simulink subsystem "Rigid_Body_Dynamics_Subsystem"  (R2026a)
settings: Solver=VariableStepAuto
settings Model: Creator=Eeman Aleem  LastModifiedBy=Eeman Aleem

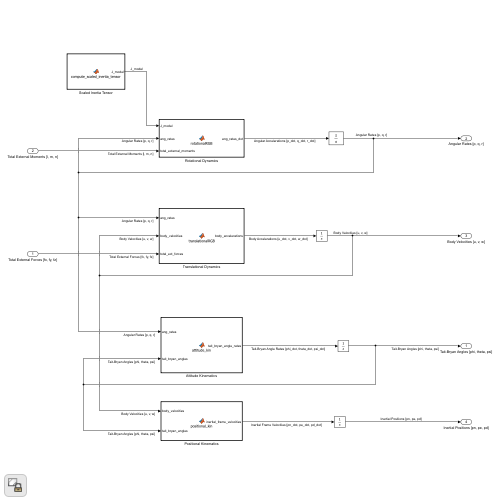
[thumbnail: Simulink's stored preview of the top-level diagram]
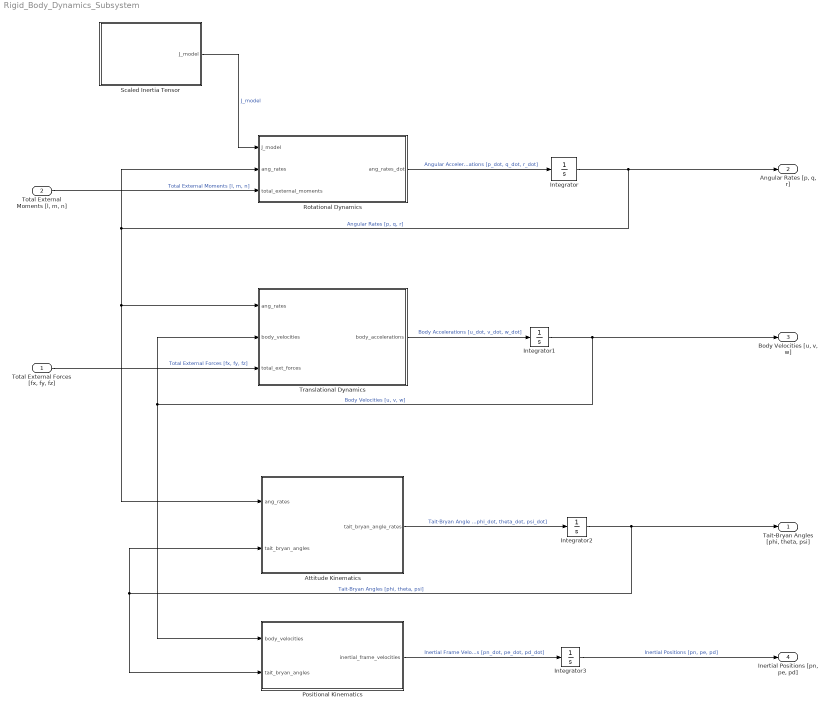
== system Rigid_Body_Dynamics_Subsystem ==
  "Total External Forces [fx, fy, fz]" : Inport
  "Total External Moments [l, m, n]" : Inport  Port=2
  Attitude Kinematics : MATLAB Function  TreatAsAtomicUnit=on
  Integrator{,1..3} (4 alike) : Integrator
  Positional Kinematics : MATLAB Function  TreatAsAtomicUnit=on
  Rotational Dynamics : MATLAB Function  TreatAsAtomicUnit=on
  Scaled Inertia Tensor : MATLAB Function  TreatAsAtomicUnit=on
  Translational Dynamics : MATLAB Function  TreatAsAtomicUnit=on
  "Tait-Bryan Angles [phi, theta, psi]" : Outport
  "Angular Rates [p, q, r]" : Outport  Port=2
  "Body Velocities [u, v, w]" : Outport  Port=3
  "Inertial Positions [pn, pe, pd]" : Outport  Port=4
  wires:
  Translational Dynamics/1(body_accelerations) -> Integrator1/1  "Body Accelerations [u_dot, v_dot, w_dot]"
  Positional Kinematics/1(inertial_frame_velocities) -> Integrator3/1  "Inertial Frame Velocities [pn_dot, pe_dot, pd_dot]"
  Rotational Dynamics/1(ang_rates_dot) -> Integrator/1  "Angular Accelerations [p_dot, q_dot, r_dot]"
  Attitude Kinematics/1(tait_bryan_angle_rates) -> Integrator2/1  "Tait-Bryan Angle Rates [phi_dot, theta_dot, psi_dot]"
  "Total External Moments [l, m, n]"/1 -> Rotational Dynamics/3(total_external_moments)  "Total External Moments [l, m, n]"
  Integrator3/1 -> "Inertial Positions [pn, pe, pd]"/1  "Inertial Positions [pn, pe, pd]"
  Integrator/1 -> Attitude Kinematics/1(ang_rates), Translational Dynamics/1(ang_rates), Rotational Dynamics/2(ang_rates), "Angular Rates [p, q, r]"/1  "Angular Rates [p, q, r]"
  Scaled Inertia Tensor/1(J_model) -> Rotational Dynamics/1(J_model)  "J_model"
  Integrator2/1 -> Attitude Kinematics/2(tait_bryan_angles), Positional Kinematics/2(tait_bryan_angles), "Tait-Bryan Angles [phi, theta, psi]"/1  "Tait-Bryan Angles [phi, theta, psi]"
  "Total External Forces [fx, fy, fz]"/1 -> Translational Dynamics/3(total_ext_forces)  "Total External Forces [fx, fy, fz]"
  Integrator1/1 -> Positional Kinematics/1(body_velocities), Translational Dynamics/2(body_velocities), "Body Velocities [u, v, w]"/1  "Body Velocities [u, v, w]"

== matlab function Rigid_Body_Dynamics_Subsystem/Rotational Dynamics ==
  data: J_model input size=[1 4]; ang_rates input size=[1 3]; ang_rates_dot output size=[1 3]; total_external_moments input size=[1 3]
function ang_rates_dot = rotationalRGB(J_model, ang_rates, total_external_moments)
    
    % Clarifying vars used
    Jx = J_model(1);
    Jy = J_model(2);
    Jz = J_model(3);
    Jxz = J_model(4);
    p = ang_rates(1);
    q = ang_rates(2);
    r = ang_rates(3);
    l = total_external_moments(1);
    m = total_external_moments(2);
    n = total_external_moments(3);
    
    % Calculate gamma constants from Equation 9
    Gamma = Jx * Jz - Jxz^2;
    Gamma1 = (Jxz * (Jx - Jy + Jz)) / Gamma;
    Gamma2 = ((Jz * (Jz - Jy)) + Jxz^2) / Gamma;
    Gamma3 = Jz / Gamma;
    Gamma4 = Jxz / Gamma;
    Gamma5 = (Jz - Jx) / Jy;
    Gamma6 = Jxz / Jy;
    Gamma7 = ((Jx * (Jx - Jy)) + Jxz^2) / Gamma;
    Gamma8 = Jx / Gamma;
    
    % Equation 9
    p_dot = Gamma1*p*q - Gamma2*q*r + Gamma3*l + Gamma4*n;
    q_dot = Gamma5*p*r - Gamma6*(p^2 - r^2) + (1/Jy)*m;
    r_dot = Gamma7*p*q - Gamma1*q*r + Gamma4*l + Gamma8*n;
    
    ang_rates_dot = [p_dot, q_dot, r_dot];

end

== matlab function Rigid_Body_Dynamics_Subsystem/Scaled Inertia Tensor ==
  data: J_model output size=[1 4]
function J_model = compute_scaled_inertia_tensor()
% This function calculates the scaled-down inertias for a model aircraft.
% It converts full-scale imperial inertias to SI units and applies a scaling factor.
%
% INPUTS:
%   J_fs array:
%       - Jx_full:   Full-scale roll inertia [slug·ft²]
%       - Jy_full:   Full-scale pitch inertia [slug·ft²]
%       - Jz_full:   Full-scale yaw inertia [slug·ft²]
%       - Jxz_full:  Full-scale product of inertia [slug·ft²]
%   mass array:
%       - m_full:    Full-scale aircraft mass [kg]
%       - m_model:   Model aircraft mass [kg]
%   gsf: Geometric scale factor
%
% OUTPUTS:
%   Jx: Scaled model roll inertia [kg·m²]
%   Jy: Scaled model pitch inertia [kg·m²]
%   Jz: Scaled model yaw inertia [kg·m²]
%   Jxz: Scaled model product of inertia [kg·m²]

% Input Constants:
m_model = GeoConsts.m_model;
m_full = GeoConsts.m_full;
gsf = GeoConsts.gsf;
J_fs = GeoConsts.J_fs;

% Unit conversion constant
slugft2_to_kgm2 = 1.35581795;

% Effective inertia scaling factor = (mass_ratio) * (length_ratio)^2
s = (m_model / m_full) * (gsf ^ 2);

% Convert full-scale inertias from imperial (slug·ft²) to SI (kg·m²)
Jx_full_SI = J_fs(1) * slugft2_to_kgm2;
Jy_full_SI = J_fs(2) * slugft2_to_kgm2;
Jz_full_SI = J_fs(3) * slugft2_to_kgm2;
Jxz_full_SI = J_fs(4) * slugft2_to_kgm2;

% Apply scaling to get the final model inertias in SI units
Jx = Jx_full_SI * s;
Jy = Jy_full_SI * s;
Jz = Jz_full_SI * s;
Jxz = Jxz_full_SI * s;

J_model = [Jx, Jy, Jz, Jxz];

end

== matlab function Rigid_Body_Dynamics_Subsystem/Translational Dynamics ==
  data: ang_rates input size=[1 3]; body_accelerations output size=[1 3]; body_velocities input size=[1 3]; total_ext_forces input size=[1 3]
function body_accelerations = translationalRGB(ang_rates, body_velocities, total_ext_forces)
    % Set up vars for clarity
    p = ang_rates(1);
    q = ang_rates(2);
    r = ang_rates(3);
    u = body_velocities(1);
    v = body_velocities(2);
    w = body_velocities(3);
    fx = total_ext_forces(1);
    fy = total_ext_forces(2);
    fz = total_ext_forces(3);
    m = GeoConsts.m_model;

    % Equation 6
    u_dot = r*v - q*w + fx/m;
    v_dot = p*w - r*u + fy/m;
    w_dot = q*u - p*v + fz/m;

    % Return body accelerations
    body_accelerations = [u_dot, v_dot, w_dot];
end

== matlab function Rigid_Body_Dynamics_Subsystem/Attitude Kinematics ==
  data: ang_rates input size=[1 3]; tait_bryan_angle_rates output size=[1 3]; tait_bryan_angles input size=[1 3]
function tait_bryan_angle_rates = attitude_kin(ang_rates, tait_bryan_angles)
    % Set up vars for clarity
    p = ang_rates(1);
    q = ang_rates(2);
    r = ang_rates(3);
    phi = tait_bryan_angles(1);
    theta = tait_bryan_angles(2);
    
    % Equation 4
    phi_dot   = p + q*sin(phi)*tan(theta) + r*cos(phi)*tan(theta);
    theta_dot = q*cos(phi) - r*sin(phi);
    psi_dot   = q*(sin(phi)/cos(theta)) + r*(cos(phi)/cos(theta));
    
    tait_bryan_angle_rates = [phi_dot, theta_dot, psi_dot];

end

== matlab function Rigid_Body_Dynamics_Subsystem/Positional Kinematics ==
  data: body_velocities input size=[1 3]; inertial_frame_velocities output size=[1 3]; tait_bryan_angles input size=[1 3]
function inertial_frame_velocities = positional_kin(body_velocities, tait_bryan_angles)

    % Set up vars for clarity
    u = body_velocities(1);
    v = body_velocities(2);
    w = body_velocities(3);
    phi = tait_bryan_angles(1);
    theta = tait_bryan_angles(2);
    psi = tait_bryan_angles(3);

    % Rotation Matrix from Equation 1 (transposed for body-to-vehicle)
    R_b_v = [cos(theta)*cos(psi), sin(phi)*sin(theta)*cos(psi) - cos(phi)*sin(psi), cos(phi)*sin(theta)*cos(psi) + sin(phi)*sin(psi);
             cos(theta)*sin(psi), sin(phi)*sin(theta)*sin(psi) + cos(phi)*cos(psi), cos(phi)*sin(theta)*sin(psi) - sin(phi)*cos(psi);
             -1*sin(theta),         sin(phi)*cos(theta),                              cos(phi)*cos(theta)];

    % Equation 3 (outputs pn_dot, pe_dot, pd_dot)
    inertial_frame_velocities_col_vector = R_b_v * [u; v; w];
    inertial_frame_velocities = [inertial_frame_velocities_col_vector(1), inertial_frame_velocities_col_vector(2), inertial_frame_velocities_col_vector(3)];
end
